simulink model "chap3_4sim"  (Simulink 5.0)
settings: Solver=ode45  StartTime=0.0  StopTime=30  RelTol=1e-5
settings Model: LastModifiedBy=Administrator  ExtModeTrigMode=oneshot  ExtModeArmWhenConnect=off  LimitDataPoints=off  BooleanDataType=off

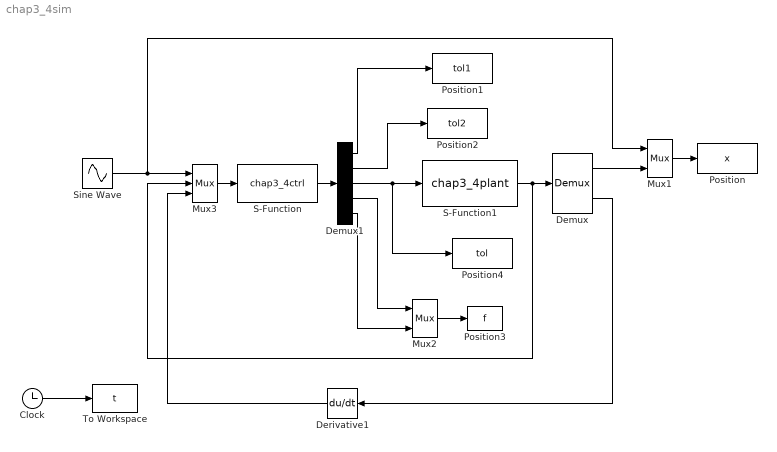
== system chap3_4sim ==
  Clock : Clock
      settings: Decimation=10
  Demux : Demux  Outputs=2
  Demux1 : Demux  Outputs=5
  Derivative1 : Derivative  Orientation=left
  Mux1 : Mux  Inputs=2
  Mux2 : Mux  Inputs=2
  Mux3 : Mux  Inputs=3
  Position : ToWorkspace  VariableName=x  SampleTime=-1  SaveFormat=Array
  Position1 : ToWorkspace  VariableName=tol1  SampleTime=-1  SaveFormat=Array
  Position2 : ToWorkspace  VariableName=tol2  SampleTime=-1  SaveFormat=Array
  Position3 : ToWorkspace  VariableName=f  SampleTime=-1  SaveFormat=Array
  Position4 : ToWorkspace  VariableName=tol  SampleTime=-1  SaveFormat=Array
  S-Function : S-Function  FunctionName=chap3_4ctrl
  S-Function1 : S-Function  FunctionName=chap3_4plant
  Sine Wave : Sin  SampleTime=0
  To Workspace : ToWorkspace  VariableName=t  SampleTime=-1  SaveFormat=Array
  wires:
  Mux1/1 -> Position/1
  Demux/1 -> Mux1/2
  Demux/2 -> Derivative1/1
  S-Function1/1 -> Demux/1, Mux3/2
  Mux3/1 -> S-Function/1
  Sine Wave/1 -> Mux3/1, Mux1/1
  Derivative1/1 -> Mux3/3
  S-Function/1 -> Demux1/1
  Demux1/3 -> S-Function1/1, Position4/1
  Demux1/1 -> Position1/1
  Demux1/2 -> Position2/1
  Mux2/1 -> Position3/1
  Demux1/4 -> Mux2/1
  Demux1/5 -> Mux2/2
  Clock/1 -> To Workspace/1
